simulink model "mod5"  (R2020b)
settings: Solver=VariableStepAuto  StartTime=0.0  StopTime=20  RelTol=1e-3
settings Model: PacingRate=20  Creator=com  LastModifiedBy=com

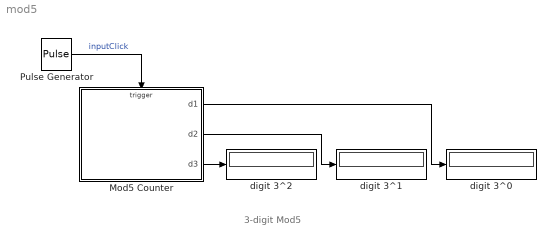
== system mod5 ==
  note: 3-digit Mod5
  Mod5 Counter : Stateflow chart  TreatAsAtomicUnit=on
  Pulse Generator : DiscretePulseGenerator  PulseType=Time based  Period=1  PulseWidth=5
  digit 3^0 : Display
  digit 3^1 : Display
  digit 3^2 : Display
  wires:
  Mod5 Counter/1(d1) -> digit 3^0/1
  Mod5 Counter/3(d3) -> digit 3^2/1
  Mod5 Counter/2(d2) -> digit 3^1/1
  Pulse Generator/1 -> Mod5 Counter/Trigger  "inputClick"

== stateflow chart mod5/Mod5 Counter ==
  settings: executeAtInitialization=1
  state digit1 [parallel]
    settings: executionOrder=1
    state two
      en:d1=2;
    state one
      en: d1 = 1;
    state zero
      en: d1 = 0;
    state three
      en:d1=3;
    state four
      en: d1 = 4;
    digit1.zero -> digit1.one : inputClick
    digit1.one -> digit1.two : inputClick
    digit1.two -> digit1.three : inputClick
    (default) -> digit1.zero
    digit1.four -> digit1.zero : inputClick /{digit2.inc2;}
    digit1.three -> digit1.four : inputClick
  state digit2 [parallel]
    settings: executionOrder=2
    state one
      en: d2 = 1;
    state two
      en:d2=2;
    state zero
      en: d2 = 0;
    state three
      en:d2=3;
    state four
      en: d2 = 4;
    digit2.zero -> digit2.one : inc2
    digit2.one -> digit2.two : inc2
    digit2.two -> digit2.three : inc2
    (default) -> digit2.zero
    digit2.four -> digit2.zero : inc2 / {digit3.inc3;}
    digit2.three -> digit2.four : inc2
  state digit3 [parallel]
    settings: executionOrder=3
    state one
      en: d3 = 1;
    state two
      en:d3=2;
    state zero
      en: d3 = 0;
    state four
      en: d3 = 4;
    state three
      en:d3=3;
    digit3.zero -> digit3.one : inc3
    digit3.one -> digit3.two : inc3
    digit3.two -> digit3.three : inc3
    (default) -> digit3.zero
    digit3.four -> digit3.zero : inc3
    digit3.three -> digit3.four : inc3
  data: d1 output int32 size=1 =0; d2 output int32 size=1 =0; d3 output int32 size=1 =0
  events: inc2 local EITHER_EDGE_EVENT; inc3 local EITHER_EDGE_EVENT; inputClick input EITHER_EDGE_EVENT
